simulink model "sim_sistema_obs_tf"  (Simulink 7.5)
settings: Solver=ode3  StartTime=0.0  StopTime=6  FixedStep=1e-4  RelTol=1e-3
values from neighbouring files (symbols this model uses):
  A = sys.a    [exemplo.m]    (also in exemplo_compara_bode.m; exemplo_compara_rlocus.m)
  B = sys.b    [exemplo.m]    (also in exemplo_compara_bode.m; exemplo_compara_rlocus.m)
  K = acker(A,B,J)    [exemplo.m]    (also in exemplo_compara_bode.m; exemplo_compara_rlocus.m)
undefined symbols (not defined in the file or in its folder): den, num
settings Model: Creator=taniel.franklin  LastModifiedBy=taniel.franklin

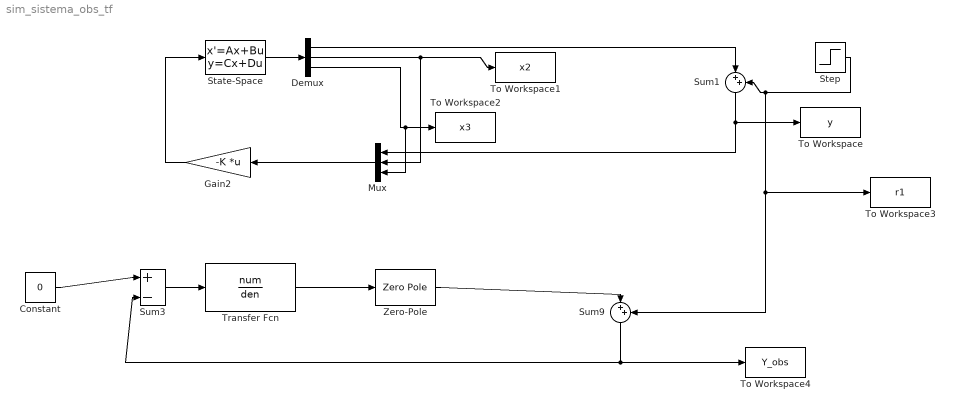
== system sim_sistema_obs_tf ==
  Constant : Constant  Value=0  OutDataType=fixdt(1, 16)  OutScaling=2^0
  Demux : Demux  Outputs=3
  Gain2 : Gain  Gain=-K  Multiplication=Matrix(K*u)  ParameterDataType=fixdt(1, 16)  ParameterScaling=2^0  OutDataType=fixdt(1, 16)  OutScaling=2^0
  Mux : Mux  Inputs=3
  State-Space : StateSpace  A=A  B=B  C=eye(3)  D=[0;0;0]
  Step : Step  Time=0.5  SampleTime=0
  Sum1 : Sum  Inputs=|++  OutDataType=fixdt(1, 16)  OutScaling=2^0
  Sum3 : Sum  Inputs=|+-  OutDataType=fixdt(1, 16)  OutScaling=2^0
  Sum9 : Sum  Inputs=|++  OutDataType=fixdt(1, 16)  OutScaling=2^0
  To Workspace : ToWorkspace  VariableName=y  SampleTime=-1  SaveFormat=Structure With Time
  To Workspace1 : ToWorkspace  VariableName=x2  SampleTime=-1  SaveFormat=Structure With Time
  To Workspace2 : ToWorkspace  VariableName=x3  SampleTime=-1  SaveFormat=Structure With Time
  To Workspace3 : ToWorkspace  VariableName=r1  SampleTime=-1  SaveFormat=Structure With Time
  To Workspace4 : ToWorkspace  VariableName=Y_obs  SampleTime=-1  SaveFormat=Structure With Time
  Transfer Fcn : TransferFcn  Numerator=num  Denominator=den
  Zero-Pole : ZeroPole  Zeros=[-2]  Poles=[0 -4 -6]  Gain=[10]
  wires:
  State-Space/1 -> Demux/1
  Demux/2 -> To Workspace1/1, Mux/2
  Gain2/1 -> State-Space/1
  Demux/1 -> Sum1/1
  Zero-Pole/1 -> Sum9/1
  Sum9/1 -> Sum3/2, To Workspace4/1
  Mux/1 -> Gain2/1
  Sum3/1 -> Transfer Fcn/1
  Constant/1 -> Sum3/1
  Transfer Fcn/1 -> Zero-Pole/1
  Demux/3 -> To Workspace2/1, Mux/3
  Sum1/1 -> Mux/1, To Workspace/1
  Step/1 -> Sum1/2, Sum9/2, To Workspace3/1
